simulink model "Mendoza2021198"  (R2024b)
settings: Solver=ode45  StartTime=0.0  StopTime=10.0  RelTol=1e-3
libraries: slpidlib x1, simulink x1
settings Model: Creator=Marco
settings DataIOCC: ReturnWorkspaceOutputs=off  TimeSaveName=t
settings DebuggingCC: AlgebraicLoopMsg=none  ArtificialAlgebraicLoopMsg=none  MaxConsecutiveZCsMsg=none  OperatingPointInterfaceChecksumMismatchMsg=none
settings RTWCC: GPUComputeCapability=3.5

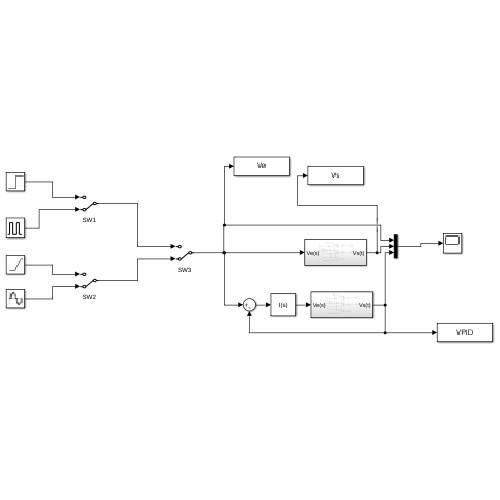
[thumbnail: Simulink's stored preview of the top-level diagram]
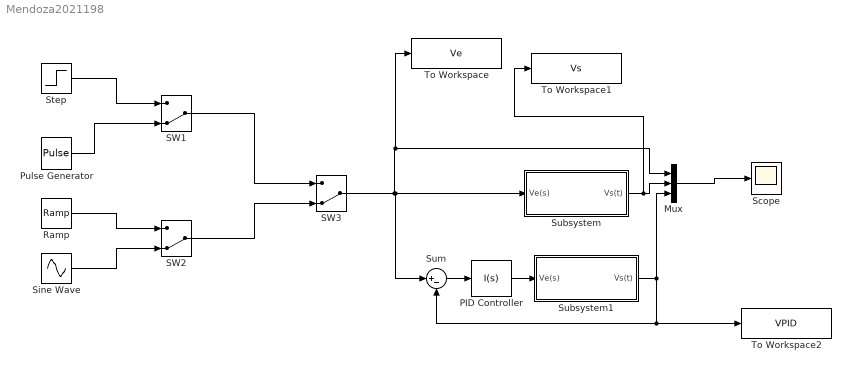
== system Mendoza2021198 ==
  Mux : Mux  Inputs=3
  PID Controller : slpidlib/PID Controller  Controller=I  Form=Parallel  TimeDomain=Continuous-time  UseExternalTs=off  SampleTime=-1  IntegratorMethod=Forward Euler  FilterMethod=Forward Euler  ControllerParametersSource=internal  P=1  I=246.2452  UseKiTs=off  D=0  UseExternalDerivativeSource=off  N=100  UseFilter=on  TunerSelectOption=Transfer Function Based (PID Tuner App)  InitialConditionSource=internal  InitialConditionForIntegrator=0  InitialConditionForFilter=0  DifferentiatorICPrevScaledInput=0  ExternalReset=none  TrackingMode=off  Kt=1  LimitOutput=off  SatLimitsSource=internal  UpperSaturationLimit=inf  LowerSaturationLimit=-inf  LinearizeAsGain=on  AntiWindupMode=none  Kb=1  LimitIntegrator=off  UpperIntegratorSaturationLimit=inf  LowerIntegratorSaturationLimit=-inf  POutMin=[]  POutMax=[]  IOutMin=[]  IOutMax=[]  DOutMin=[]  DOutMax=[]  NOutMin=[]  NOutMax=[]  SumOutMin=[]  SumOutMax=[]  SaturationOutMin=[]  SaturationOutMax=[]  PParamMin=[]  PParamMax=[]  IParamMin=[]  IParamMax=[]  DParamMin=[]  DParamMax=[]  NParamMin=[]  NParamMax=[]  KbParamMin=[]  KbParamMax=[]  KtParamMin=[]  KtParamMax=[]  KbOutMin=[]  KbOutMax=[]  KtOutMin=[]  KtOutMax=[]  IntegratorOutMin=[]  IntegratorOutMax=[]  FilterOutMin=[]  FilterOutMax=[]  SumI1OutMin=[]  SumI1OutMax=[]  SumI2OutMin=[]  SumI2OutMax=[]  SumI3OutMin=[]  SumI3OutMax=[]  SumI4OutMin=[]  SumI4OutMax=[]  SumDOutMin=[]  SumDOutMax=[]  DifferentiatorOutMin=[]  DifferentiatorOutMax=[]  FilterDiffOutCoefMin=[]  FilterDiffOutCoefMax=[]  ReciprocalOutMin=[]  ReciprocalOutMax=[]  SumDenOutMin=[]  SumDenOutMax=[]  SumNumOutMin=[]  SumNumOutMax=[]  DivideOutMin=[]  DivideOutMax=[]  UdiffTsProdOutMin=[]  UdiffTsProdOutMax=[]  NTsProdOutMin=[]  NTsProdOutMax=[]  UintegralTsProdOutMin=[]  UintegralTsProdOutMax=[]  UngainTsProdOutMin=[]  UngainTsProdOutMax=[]  ClampingZeroOutDataTypeStr=Inherit: Inherit via back propagation  ClampingZeroOutMin=[]  ClampingZeroOutMax=[]  FilterDenConstantOutDataTypeStr=Inherit: Inherit via back propagation  FilterDenConstantOutMin=[]  FilterDenConstantOutMax=[]  PCopyOutDataTypeStr=Inherit: Inherit via back propagation  PCopyOutMin=[]  PCopyOutMax=[]  NCopyOutDataTypeStr=Inherit: Inherit via back propagation  NCopyOutMin=[]  NCopyOutMax=[]  IntegratorContinuousStateAttributes=''  IntegratorStateMustResolveToSignalObject=off  IntegratorRTWStateStorageClass=Auto  FilterContinuousStateAttributes=''  FilterStateMustResolveToSignalObject=off  FilterRTWStateStorageClass=Auto  ParallelPVariant=Disabled  IdealPVariant=Disabled  IVariant=InternalParameters  DVariant=Disabled  IntegratorVariant=Continuous  SatVariant=Disabled  AWVariant=Passthrough  PCopyVariant=Disabled  TRVariant=Disabled  FdbkBlocksVariant=Forward  IdealPFdbkVariant=Disabled  SatFdbkVariant=Disabled  DerivativeFilterVariant=Disabled  NVariant=Disabled  NCopyVariant=Disabled_SignalSpec  FilterICVariant=Disabled  IntegratorICVariant=InternalICs  ExternalResetVariant=Disabled  TRSumVariant=Passthrough  SumFdbkVariant=Disabled  SumVariant=Passthrough_I  TsampFilterVariant=InternalTs  TsampNgainVariant=Passthrough  TsampIntegralVariant=Disabled_SignalSpec  ExternalSaturationOutDataTypeStr=Inherit: Same as second input  DerivativeSourceVariant=Disabled  PreIntVariant=InternalPreInt
  Pulse Generator : DiscretePulseGenerator  PulseType=Time based  Period=10  PulseWidth=10  PhaseDelay=1
  Ramp : simulink/Sources/Ramp  slope=1/10  start=0  InitialOutput=0
  SW1 : ManualSwitch  CurrentSetting=0
  SW2 : ManualSwitch  CurrentSetting=0
  SW3 : ManualSwitch  CurrentSetting=0
  Scope : Scope
  Sine Wave : Sin  Frequency=1.5708  SampleTime=0.001
  Step : Step  Time=0  SampleTime=0.001
  Subsystem : Subsystem
  Subsystem1 : Subsystem
  Sum : Sum  Inputs=|+-
  To Workspace : ToWorkspace  VariableName=Ve  SampleTime=-1
  To Workspace1 : ToWorkspace  VariableName=Vs  SampleTime=-1
  To Workspace2 : ToWorkspace  VariableName=VPID  SampleTime=-1
  wires:
  Step/1 -> SW1/1
  Pulse Generator/1 -> SW1/2
  Ramp/1 -> SW2/1
  SW2/1 -> SW3/2
  SW1/1 -> SW3/1
  SW3/1 -> Sum/1, Subsystem/1(Ve(s)), To Workspace/1, Mux/1
  Subsystem/1(Vs(t)) -> To Workspace1/1, Mux/2
  Mux/1 -> Scope/1
  PID Controller/1 -> Subsystem1/1(Ve(s))
  Sum/1 -> PID Controller/1
  Subsystem1/1(Vs(t)) -> Sum/2, To Workspace2/1, Mux/3
  Sine Wave/1 -> SW2/2

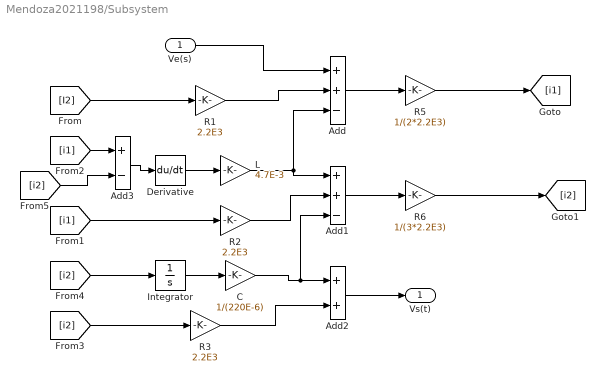
== system Mendoza2021198/Subsystem ==
  Ve(s) : Inport
  Add : Sum  Inputs=++-
  Add1 : Sum  Inputs=++-
  Add2 : Sum
  Add3 : Sum  Inputs=+-
  C : Gain  Gain=1/(220E-6)
  Derivative : Derivative
  Integrator : Integrator
  L : Gain  Gain=4.7E-3
  R1 : Gain  Gain=2.2E3
  R2 : Gain  Gain=2.2E3
  R3 : Gain  Gain=2.2E3
  R5 : Gain  Gain=1/(2*2.2E3)
  R6 : Gain  Gain=1/(3*2.2E3)
  Vs(t) : Outport
  wires:
  Ve(s)/1 -> Add/1
  [I2] -> R1/1
  R1/1 -> Add/2
  Derivative/1 -> L/1
  L/1 -> Add/3, Add1/1
  R2/1 -> Add1/2
  [i1] -> R2/1
  C/1 -> Add1/3, Add2/1
  Integrator/1 -> C/1
  [i2] -> Integrator/1
  [i1] -> Add3/1
  [i2] -> Add3/2
  [i2] -> R3/1
  R3/1 -> Add2/2
  Add2/1 -> Vs(t)/1
  Add1/1 -> R6/1
  Add/1 -> R5/1
  R5/1 -> [i1]
  R6/1 -> [i2]
  Add3/1 -> Derivative/1

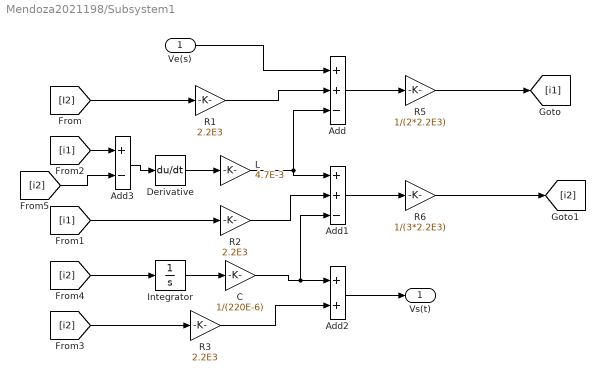
== system Mendoza2021198/Subsystem1 ==
  Ve(s) : Inport
  Add : Sum  Inputs=++-
  Add1 : Sum  Inputs=++-
  Add2 : Sum
  Add3 : Sum  Inputs=+-
  C : Gain  Gain=1/(220E-6)
  Derivative : Derivative
  Integrator : Integrator
  L : Gain  Gain=4.7E-3
  R1 : Gain  Gain=2.2E3
  R2 : Gain  Gain=2.2E3
  R3 : Gain  Gain=2.2E3
  R5 : Gain  Gain=1/(2*2.2E3)
  R6 : Gain  Gain=1/(3*2.2E3)
  Vs(t) : Outport
  wires:
  Ve(s)/1 -> Add/1
  [I2] -> R1/1
  R1/1 -> Add/2
  Derivative/1 -> L/1
  L/1 -> Add/3, Add1/1
  R2/1 -> Add1/2
  [i1] -> R2/1
  C/1 -> Add1/3, Add2/1
  Integrator/1 -> C/1
  [i2] -> Integrator/1
  [i1] -> Add3/1
  [i2] -> Add3/2
  [i2] -> R3/1
  R3/1 -> Add2/2
  Add2/1 -> Vs(t)/1
  Add1/1 -> R6/1
  Add/1 -> R5/1
  R5/1 -> [i1]
  R6/1 -> [i2]
  Add3/1 -> Derivative/1
